simulink model "dianrong_luenbege"  (R2023b)
settings: Solver=VariableStepAuto  StartTime=0.0  StopTime=10.0  RelTol=1e-3
settings Model: Creator=CSC  LastModifiedBy=CSC

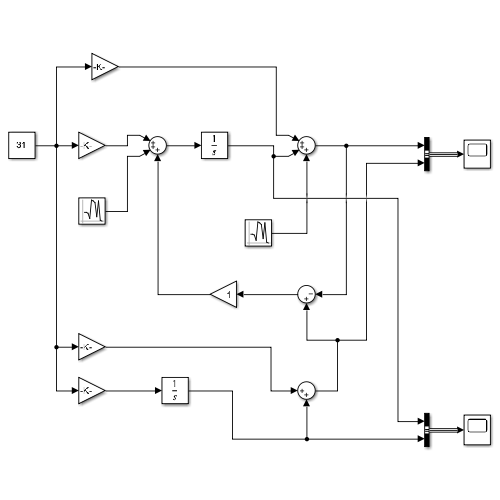
[thumbnail: Simulink's stored preview of the top-level diagram]
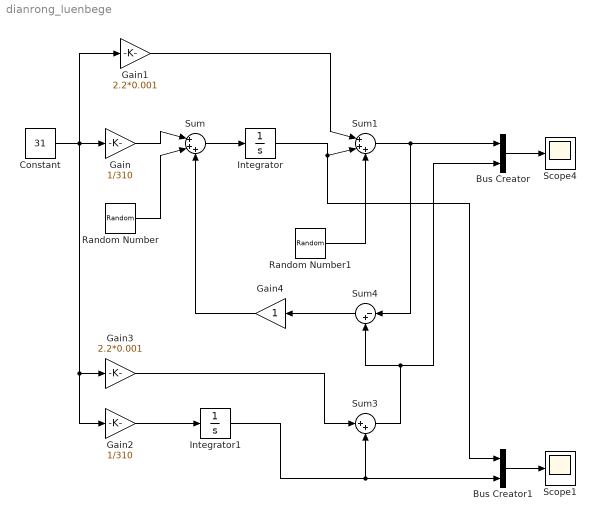
== system dianrong_luenbege ==
  Bus Creator : BusCreator  Inputs=2
  Bus Creator1 : BusCreator  Inputs=2
  Constant : Constant  Value=31
  Gain : Gain  Gain=1/310
  Gain1 : Gain  Gain=2.2*0.001
  Gain2 : Gain  Gain=1/310
  Gain3 : Gain  Gain=2.2*0.001
  Gain4 : Gain
  Integrator : Integrator
  Integrator1 : Integrator
  Random Number : RandomNumber  Variance=0.01  SampleTime=0.1
  Random Number1 : RandomNumber  Variance=0.01  SampleTime=0.1
  Scope1 : Scope
  Scope4 : Scope
  Sum : Sum  Inputs=|+++
  Sum1 : Sum  Inputs=|+++
  Sum3 : Sum  Inputs=|++
  Sum4 : Sum  Inputs=|-+
  wires:
  Sum/1 -> Integrator/1
  Constant/1 -> Gain2/1, Gain3/1, Gain/1, Gain1/1
  Gain/1 -> Sum/1
  Sum1/1 -> Sum4/1, Bus Creator/1
  Integrator/1 -> Bus Creator1/1, Sum1/2
  Gain1/1 -> Sum1/1
  Random Number/1 -> Sum/2
  Random Number1/1 -> Sum1/3
  Gain2/1 -> Integrator1/1
  Gain3/1 -> Sum3/1
  Sum3/1 -> Sum4/2, Bus Creator/2
  Integrator1/1 -> Bus Creator1/2, Sum3/2
  Sum4/1 -> Gain4/1
  Bus Creator/1 -> Scope4/1
  Bus Creator1/1 -> Scope1/1
  Gain4/1 -> Sum/3
